simulink model "operationalSpacePDControl"  (R2021a)
settings: Solver=VariableStepAuto  StartTime=0.0  StopTime=15  RelTol=1e-3
values from neighbouring files (symbols this model uses):
  Kd = diag([20, 20, 20, 10, 10, 10])    [assignment9_main.m]
  Kp = diag([30, 30, 30, 20,20, 20])    [assignment9_main.m]
  x_d = goalPose_0    [assignment9_main.m]
libraries: vrlib x1
settings Model: Creator=fabio  LastModifiedBy=fabio
settings DebuggingCC: UnconnectedInputMsg=none  UnconnectedOutputMsg=none

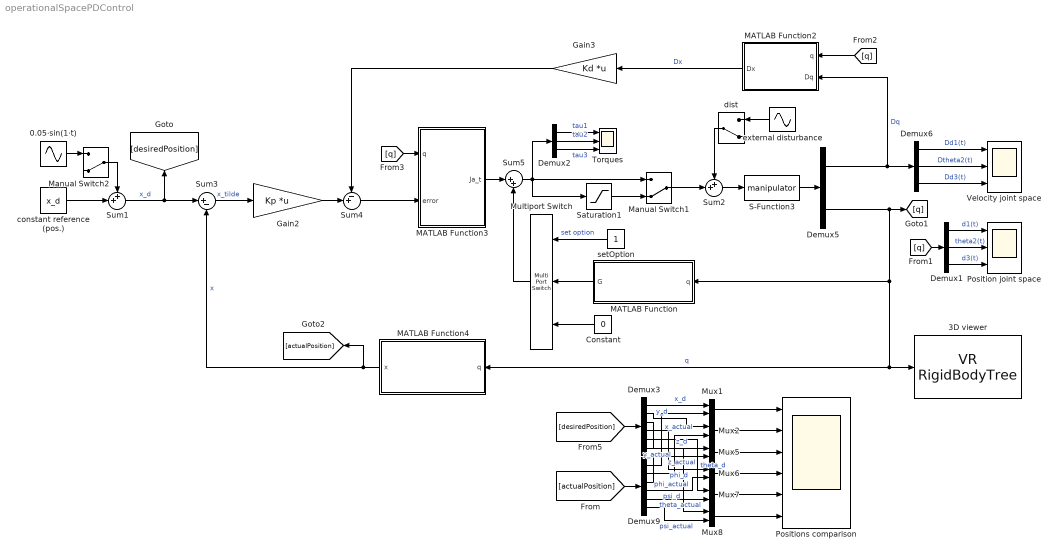
== system operationalSpacePDControl ==
  "0.05·sin(1·t) " : Sin  Amplitude=0.05  SampleTime=0
  3D viewer : vrlib/VR RigidBodyTree  RBT=robot  useRBT=off  Ts=0.5  ForceViewerOpen=on
      settings: SourceProductBaseCode=SL
  Constant : Constant  Value=0
  Demux1 : Demux  Outputs=3
  Demux2 : Demux  Outputs=3
  Demux3 : Demux  Outputs=6
  Demux5 : Demux  Outputs=2
  Demux6 : Demux  Outputs=3
  Demux9 : Demux  Outputs=6
  Gain2 : Gain  Gain=Kp  Multiplication=Matrix(K*u) (u vector)
  Gain3 : Gain  Gain=Kd  Multiplication=Matrix(K*u) (u vector)
  MATLAB Function : MATLAB Function  TreatAsAtomicUnit=on
  MATLAB Function2 : MATLAB Function  TreatAsAtomicUnit=on
  MATLAB Function3 : MATLAB Function  TreatAsAtomicUnit=on
  MATLAB Function4 : MATLAB Function  TreatAsAtomicUnit=on
  Manual Switch1 : ManualSwitch  CurrentSetting=0
  Manual Switch2 : ManualSwitch  CurrentSetting=0
  Multiport Switch : MultiPortSwitch  Inputs=2
  Mux{1..2,5..8} (6 alike) : Mux  Inputs=2
  Position joint space : Scope  NumInputPorts=3
  Positions comparison : Scope  NumInputPorts=6
  S-Function3 : S-Function  FunctionName=manipulator  Parameters=myRobot  SFunctionDeploymentMode=off  EnableBusSupport=off
  Saturation1 : Saturate  UpperLimit=10  LowerLimit=-10
  Sum1 : Sum  Inputs=++|
  Sum2 : Sum  Inputs=++|
  Sum3 : Sum  Inputs=|+-
  Sum4 : Sum  Inputs=-+|
  Sum5 : Sum  Inputs=|++
  Torques : Scope  NumInputPorts=3
  Velocity joint space : Scope  NumInputPorts=3
  constant reference (pos.) : Constant  Value=x_d
  dist : ManualSwitch  CurrentSetting=0
  external disturbance : Sin  Amplitude=0.1  SampleTime=0
  setOption : Constant
  wires:
  Sum5/1 -> Saturation1/1, Demux2/1, Manual Switch1/1
  Demux9/3 -> Mux5/2  "z_actual"
  Sum3/1 -> Gain2/1  "x_tilde"
  Sum1/1 -> Sum3/1, [desiredPosition]  "x_d"
  Demux6/3 -> Velocity joint space/3  "Dd3(t)"
  Demux6/2 -> Velocity joint space/2  "Dtheta2(t)"
  Demux6/1 -> Velocity joint space/1  "Dd1(t)"
  S-Function3/1 -> Demux5/1
  Gain3/1 -> Sum4/1
  Gain2/1 -> Sum4/2
  Multiport Switch/1 -> Sum5/2
  MATLAB Function/1(G) -> Multiport Switch/2
  Constant/1 -> Multiport Switch/3
  setOption/1 -> Multiport Switch/1  "set option"
  Demux5/1 -> MATLAB Function2/2(Dq), Demux6/1  "Dq"
  Demux5/2 -> [q], MATLAB Function4/1(q), 3D viewer/1, MATLAB Function/1(q)  "q"
  constant reference (pos.)/1 -> Sum1/2
  Demux2/1 -> Torques/1  "tau1"
  Demux2/2 -> Torques/2  "tau2"
  Demux2/3 -> Torques/3  "tau3"
  Sum2/1 -> S-Function3/1
  external disturbance/1 -> dist/1
  dist/1 -> Sum2/1
  "0.05·sin(1·t) "/1 -> Manual Switch2/1
  Manual Switch2/1 -> Sum1/1
  [actualPosition] -> Demux9/1
  MATLAB Function2/1(Dx) -> Gain3/1  "Dx"
  [q] -> MATLAB Function2/1(q)
  Sum4/1 -> MATLAB Function3/2(error)
  MATLAB Function3/1(Ja_t) -> Sum5/1
  MATLAB Function4/1(x) -> Sum3/2, [actualPosition]  "x"
  [desiredPosition] -> Demux3/1
  Demux3/3 -> Mux5/1  "z_d"
  Saturation1/1 -> Manual Switch1/2
  Manual Switch1/1 -> Sum2/2
  [q] -> Demux1/1
  Demux1/1 -> Position joint space/1  "d1(t)"
  Demux1/2 -> Position joint space/2  "theta2(t)"
  Demux1/3 -> Position joint space/3  "d3(t)"
  Demux3/1 -> Mux1/1  "x_d"
  Demux9/1 -> Mux1/2  "x_actual"
  Demux3/2 -> Mux2/1  "y_d"
  Demux9/2 -> Mux2/2  "y_actual"
  Demux3/4 -> Mux6/1  "phi_d"
  Demux9/4 -> Mux6/2  "phi_actual"
  Demux9/5 -> Mux7/2  "theta_actual"
  Demux3/5 -> Mux7/1  "theta_d"
  Demux3/6 -> Mux8/1  "psi_d"
  Demux9/6 -> Mux8/2  "psi_actual"
  Mux1/1 -> Positions comparison/1
  Mux2/1 -> Positions comparison/2
  Mux5/1 -> Positions comparison/3
  Mux6/1 -> Positions comparison/4
  Mux7/1 -> Positions comparison/5
  Mux8/1 -> Positions comparison/6
  [q] -> MATLAB Function3/1(q)

== matlab function operationalSpacePDControl/MATLAB Function ==
  data: q input; G output
function G = gravityTerm(q) 
    G = get_G_matrix(q);
end

== matlab function operationalSpacePDControl/MATLAB Function2 ==
  data: q input; Dx output; Dq input
function Dx = Ja_x_Dq(q, Dq)
    if size(q,1) < 3
        q = [0 0 0];   
    end  
    Ja = get_Ja_matrix(q);      
    Dx = Ja * Dq;
end

== matlab function operationalSpacePDControl/MATLAB Function3 ==
  data: q input; Ja_t output; error input
function Ja_t = Ja_transposed(q, error)
    %Compute the numerical analytical jacobian
    if size(q,1) < 3
        q = [0 0 0];   
    end
    
    Ja = get_Ja_matrix(q);
    Ja_t = Ja.' * error;
      
end

== matlab function operationalSpacePDControl/MATLAB Function4 ==
  data: q input; x output
function x = k(q) 
    %Compute the direct kinematics from last transformation matrix
    if size(q,1) < 3
        q = [0 0 0];   
    end
    
    %get rotation matrix and translation vector from ∑0 to ∑ee   
    T0_to_ee = get_T0_ee_matrix(q);
    R0_to_ee = T0_to_ee(1:3,1:3);
    p0_to_ee = T0_to_ee(1:3,4);    
                 
    eulerAngles = rotm2eul(R0_to_ee, 'ZYZ');
  
    x = [ p0_to_ee;
          eulerAngles.' ]; %return complete direct kinematics
    
end
